simulink model "BT"  (R2017b)
settings: Solver=ode5  StartTime=0.0  StopTime=60  FixedStep=0.1  RelTol=1e-3
libraries: fuzblock x1, powerlib_meascontrol x1
settings Model: Creator=phamt  LastModifiedBy=phamt

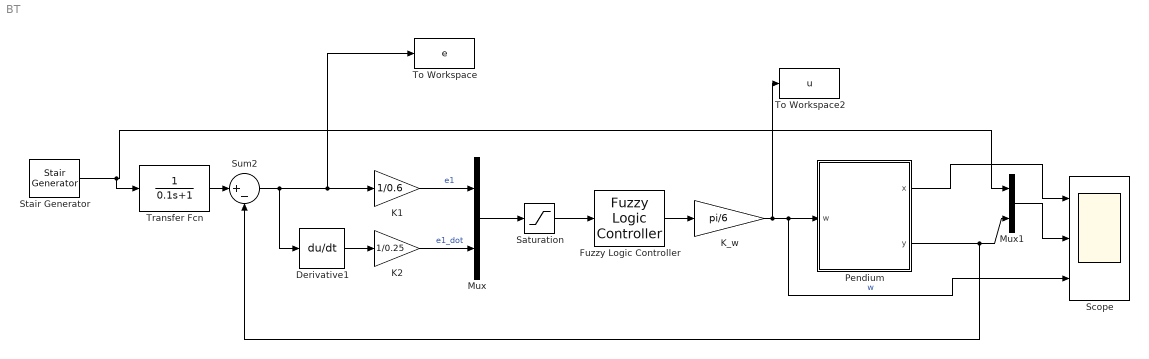
== system BT ==
  Derivative1 : Derivative
  Fuzzy Logic Controller : fuzblock/Fuzzy Logic  Controller  FIS='BT.fis'  OutputSampleNumber=101  DataType=double  FuzzifiedInputs=off  RuleFiringStrengths=off  RuleOutputs=off  AggregatedOutputs=off  SimulateUsing=Interpreted execution
  K1 : Gain  Gain=1/0.6
  K2 : Gain  Gain=1/0.25
  K_w : Gain  Gain=pi/6
  Mux : Mux  Inputs=2
  Mux1 : Mux  Inputs=2
  Pendium : Subsystem
  Saturation : Saturate  UpperLimit=1  LowerLimit=-1
  Scope : Scope  NumInputPorts=3
  Stair Generator : powerlib_meascontrol/Pulse & Signal Generators/Stair Generator  t=[0, 10, 20, 30, 40, 50, 60]  e=[0.4, 0.2, 0, 0.6, 0.2, 0.4, 0]  Ts=0
      settings: SourceProductName=Simscape Power Systems
  Sum2 : Sum  Inputs=|+-
  To Workspace : ToWorkspace  VariableName=e  SampleTime=-1
  To Workspace2 : ToWorkspace  VariableName=u  SampleTime=-1
  Transfer Fcn : TransferFcn  Denominator=[0.1 1]
  wires:
  Stair Generator/1 -> Transfer Fcn/1, Mux1/1
  K_w/1 -> To Workspace2/1, Scope/3, Pendium/1(w)  "w"
  Saturation/1 -> Fuzzy Logic Controller/1
  Fuzzy Logic Controller/1 -> K_w/1
  Mux1/1 -> Scope/2
  Pendium/2(y) -> Mux1/2, Sum2/2
  K1/1 -> Mux/1  "e1"
  Sum2/1 -> Derivative1/1, To Workspace/1, K1/1
  Mux/1 -> Saturation/1
  Derivative1/1 -> K2/1
  K2/1 -> Mux/2  "e1_dot"
  Pendium/1(x) -> Scope/1
  Transfer Fcn/1 -> Sum2/1

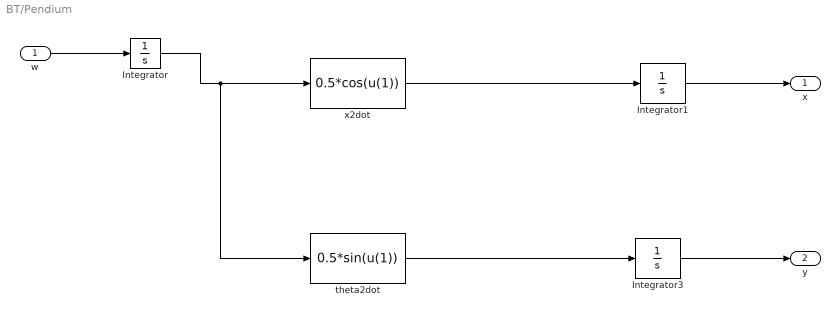
== system BT/Pendium ==
  w : Inport
  Integrator : Integrator
  Integrator1 : Integrator
  Integrator3 : Integrator
  theta2dot : Fcn  Expr=0.5*sin(u(1))
  x2dot : Fcn  Expr=0.5*cos(u(1))
  x : Outport
  y : Outport  Port=2
  wires:
  Integrator/1 -> theta2dot/1, x2dot/1
  Integrator1/1 -> x/1
  Integrator3/1 -> y/1
  x2dot/1 -> Integrator1/1
  theta2dot/1 -> Integrator3/1
  w/1 -> Integrator/1
